simulink model "znpk_example"  (R2023b)
settings: Solver=VariableStepAuto  StartTime=0.0  StopTime=200  RelTol=1e-3
settings Model: Creator=test  LastModifiedBy=Andrea
settings SolverCC: AlgebraicLoopSolver=TrustRegion
settings DebuggingCC: UnconnectedInputMsg=warning  UnconnectedOutputMsg=warning  UnconnectedLineMsg=warning
settings ModelReferenceCC: EnableRefExpFcnMdlSchedulingChecks=on
settings RTWCC: DLArmComputeVersion=19.05

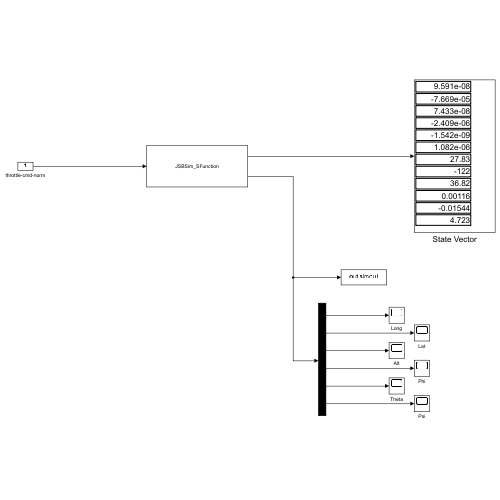
[thumbnail: Simulink's stored preview of the top-level diagram]
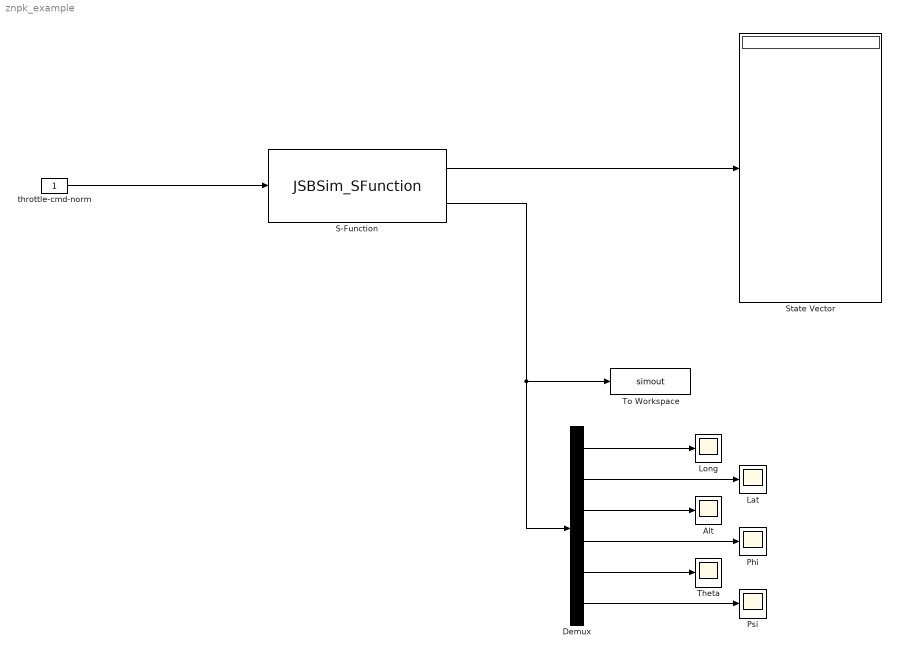
== system znpk_example ==
  Alt : Scope
  Demux : Demux  Outputs=6
  Lat : Scope
  Long : Scope
  Phi : Scope
  Psi : Scope
  S-Function : S-Function  FunctionName=JSBSim_SFunction  Parameters='ZNP-K', 0.0083333, 1, 'scripts/ZNP-K/ZNP-K-2', 'reset01', 'znpk_io'  SFunctionDeploymentMode=off  EnableBusSupport=off
  State Vector : Display
  Theta : Scope
  To Workspace : ToWorkspace  VariableName=simout  SaveFormat=Timeseries  SampleTime=-1
  throttle-cmd-norm : Constant
  wires:
  throttle-cmd-norm/1 -> S-Function/1
  S-Function/1 -> State Vector/1
  S-Function/2 -> Demux/1, To Workspace/1
  Demux/1 -> Long/1
  Demux/2 -> Lat/1
  Demux/3 -> Alt/1
  Demux/5 -> Theta/1
  Demux/4 -> Phi/1
  Demux/6 -> Psi/1
